simulink model "osek_apis"  (Simulink 6.0)
settings: Solver=FixedStepDiscrete  StartTime=0.0  StopTime=10.0  RelTol=1e-3
undefined symbols (not defined in the file or in its folder): D4, D5, green, red
libraries: oseklib x5, simulink x3, osekdrivers x2
settings Model: Creator=jcarrick  LastModifiedBy=jcarrick  ProdHWDeviceType=Motorola PowerPC
settings SolverCC: PositivePriorityOrder=on
settings DataIOCC: SignalLoggingName=sigsOut
settings OptimizationCC: InlineParams=on  InlineInvariantSignals=off  OptimizeModelRefInitCode=on  LifeSpan=1
settings DebuggingCC: CheckExecutionContextPreStartOutputMsg=on  CheckExecutionContextRuntimeOutputMsg=on  SolverPrmCheckMsg=none
settings HardwareCC: ProdEndianess=BigEndian  ProdHWDeviceType=Motorola PowerPC
settings RTWCC: SystemTargetFile=osekworks.tlc  GenCodeOnly=on  TemplateMakefile=osek_default_tmf  GenerateReport=on  RetainRTWFile=on  ProcessScript=osekworks_make_rtw_hook  IncludeHyperlinkInReport=on  LaunchReport=on
settings CodeAppCC: IgnoreCustomStorageClasses=off
settings STFCustomTargetCC: TargetFcnLib=ansi_tfl_tmw.mat  GenFloatMathFcnCalls=ANSI_C  ModelReferenceCompliant=off  CombineOutputUpdateFcns=on  SuppressErrorStatus=on  ERTCustomFileBanners=on  SystemTargetFile=osekworks.tlc  ForcedBaseTarget=off
settings ERTTargetCC: TargetFcnLib=ansi_tfl_tmw.mat  GenFloatMathFcnCalls=ANSI_C  ModelReferenceCompliant=off  SuppressErrorStatus=on  SupportContinuousTime=on  SupportNonInlinedSFcns=on  RootIOFormat=Individual Arguments  ERTCustomFileTemplate=osek_file_process.tlc  InitialValueSource=Model
settings CustomProperty: DataType=RTWOptions_EnumType__toolbox_rtw_targets_osek_osek_osekworks_bspName  Value=phycore555
settings EnumStrPairs: String=axiomcmd565
settings SFSimCC: SFSimApplyToAllLibs=on  SFSimBuildMode=Incremental

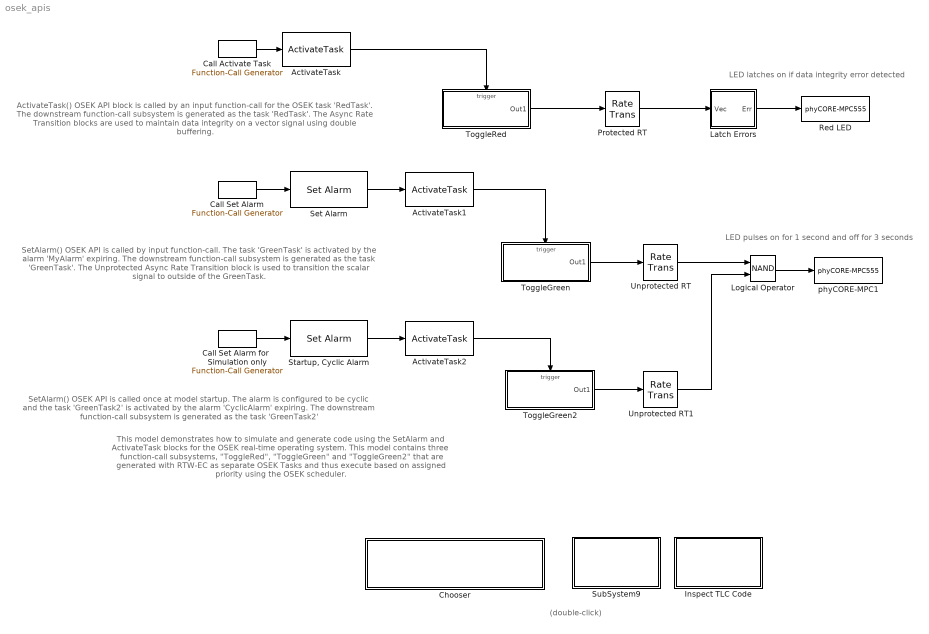
== system osek_apis ==
  note: This model demonstrates how to simulate and generate code using the SetAlarm and ActivateTask blocks
      | for the OSEK real-time operating system. This model contains three function-call subsystems, "ToggleRed",
      | "ToggleGreen" and "ToggleGreen2" that are generated with RTW-EC as separate OSEK Tasks and thus
      | execute based on assigned priority using the OSEK scheduler.
  note: (double-click)
  note: ActivateTask() OSEK API block is called by an input
      | function-call for the OSEK task 'RedTask'. The downstream
      | function-call subsystem is generated as the task 'RedTask'.
      | The Async Rate Transition blocks are used to maintain
      | data integrity on a vector signal using double buffering.
  note: SetAlarm() OSEK API is called by input function-call. The task
      | 'GreenTask' is activated by the alarm 'MyAlarm' expiring. The
      | downstream function-call subsystem is generated as the task 'GreenTask'.
      | The Unprotected Async Rate Transition block is used to transition the
      | scalar signal to outside of the GreenTask.
  note: SetAlarm() OSEK API is called once at model startup. The alarm
      | is configured to be cyclic and the task 'GreenTask2' is activated by
      | the alarm 'CyclicAlarm' expiring. The downstream function-call
      | subsystem is generated as the task 'GreenTask2'
  note: LED pulses on for 1 second and off for 3 seconds
  note: LED latches on if data integrity error detected
  ActivateTask : oseklib/ActivateTask  taskName=RedTask  taskPriority=10  taskStackSize=1000  taskSchedule=FULL
  ActivateTask1 : oseklib/ActivateTask  taskName=GreenTask  taskPriority=31  taskStackSize=100  taskSchedule=NON
  ActivateTask2 : oseklib/ActivateTask  taskName=GreenTask2  taskPriority=32  taskStackSize=100  taskSchedule=NON
  Call Activate Task : simulink/Ports & Subsystems/Function-Call Generator  sample_time=1  numberOfIterations=1
  Call Set Alarm : simulink/Ports & Subsystems/Function-Call Generator  sample_time=1  numberOfIterations=1
  Call Set Alarm for  Simulation only : simulink/Ports & Subsystems/Function-Call Generator  sample_time=2  numberOfIterations=1
  Chooser : Subsystem  LoadFcn=|  PropExecContextAcrossSSBoundary=on  mask{stf=osekworks.tlc}
      | x = osek.prefs.load('osek');                               
      | Implementation = lower(x.Implementation);                  
      | clear x;                                                   
      | switch Implementation                                      
      |  case {'proosek','osekworks'}                              
      |   osek_choose_imp([Implementation,'.tlc']);                
      |   set_param(gcb,'MaskValueString',[Implementation,'.tlc']);
      |  otherwise                                                 
      |   error(['Unrecognized implementation: ' Implementation]); 
      | end                                                        
      | clear Implementation;
      mask prompts: stf "Implementation"
      mask help: Choose OSEK System Target File
      mask init:
      | osek_choose_imp(stf)
      mask StyleString: popup(osekworks.tlc|proosek.tlc)
      mask Display: disp(['Choose System Target File:\nCurrently set to "' strtok(get_param(gcs,'rtwsystemtargetfile')) '"'])
  Inspect TLC Code : Subsystem  PropExecContextAcrossSSBoundary=on
      mask Display: disp('Inspect\nBlock\nTLC Code')
  Latch Errors : Subsystem  TreatAsAtomicUnit=on  PropExecContextAcrossSSBoundary=on
      settings: RTWSystemCode=Function
  Logical Operator : Logic  Operator=NAND  AllPortsSameDT=off
  Protected RT : RateTransition  Deterministic=off  OutPortSampleTime=.25
  Red LED : osekdrivers/phyCORE-MPC555  ledChoice=D4(red)
  Set Alarm : oseklib/Set Alarm  alarmName=MyAlarm  alarmIncr=1  alarmType=Relative  alarmPlacement=off  alarmCyclic=0
  "Startup, Cyclic Alarm" : oseklib/Set Alarm  alarmName=cyclicAlarm  alarmIncr=1  alarmType=Relative  alarmPlacement=on  alarmCyclic=8
  SubSystem9 : Subsystem  PropExecContextAcrossSSBoundary=on
      settings: OpenFcn=rtwbuild('osek_apis');
      mask Display: disp('Generate\nCode')
  ToggleGreen : Subsystem  TreatAsAtomicUnit=on  PropExecContextAcrossSSBoundary=on
      settings: RTWSystemCode=Function
  ToggleGreen2 : Subsystem  TreatAsAtomicUnit=on  PropExecContextAcrossSSBoundary=on
      settings: RTWSystemCode=Function
  ToggleRed : Subsystem  TreatAsAtomicUnit=on  PropExecContextAcrossSSBoundary=on
      settings: RTWSystemCode=Function
  Unprotected RT : RateTransition  Integrity=off  OutPortSampleTime=1
  Unprotected RT1 : RateTransition  Integrity=off  OutPortSampleTime=1
  phyCORE-MPC1 : osekdrivers/phyCORE-MPC555  ledChoice=D5(green)
  wires:
  ActivateTask/1 -> ToggleRed/Trigger
  ToggleRed/1(Out1) -> Protected RT/1
  Call Activate Task/1 -> ActivateTask/1
  Latch Errors/1(Err) -> Red LED/1
  Protected RT/1 -> Latch Errors/1(Vec)
  Set Alarm/1 -> ActivateTask1/1
  Call Set Alarm/1 -> Set Alarm/1
  ActivateTask1/1 -> ToggleGreen/Trigger
  ToggleGreen/1(Out1) -> Unprotected RT/1
  "Startup, Cyclic Alarm"/1 -> ActivateTask2/1
  Call Set Alarm for  Simulation only/1 -> "Startup, Cyclic Alarm"/1
  ActivateTask2/1 -> ToggleGreen2/Trigger
  ToggleGreen2/1(Out1) -> Unprotected RT1/1
  Unprotected RT/1 -> Logical Operator/1
  Unprotected RT1/1 -> Logical Operator/2
  Logical Operator/1 -> phyCORE-MPC1/1

== system osek_apis/Chooser ==

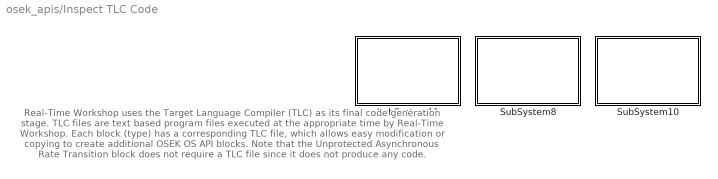
== system osek_apis/Inspect TLC Code ==
  note: Real-Time Workshop uses the Target Language Compiler (TLC) as its final code generation stage.
      | TLC files are text based program files executed at the appropriate time by Real-Time Workshop.
      | Each block (type) has a corresponding TLC file, which allows easy modification or copying to create
      | additional OSEK OS API blocks. Note that the Unprotected Asynchronous Rate Transition block does
      | not require a TLC file since it does not produce any code.
  SubSystem10 : Subsystem  PropExecContextAcrossSSBoundary=on
      settings: OpenFcn=edit(fullfile(matlabroot,'toolbox','rtw','targets','osek','blocks','osekdbuffer.tlc'));
      mask Display: disp('Inspect\nAsync Rate\nTransition\nTLC File')
  SubSystem11 : Subsystem  PropExecContextAcrossSSBoundary=on
      settings: OpenFcn=edit(fullfile(matlabroot,'toolbox','rtw','targets','osek','blocks','osektask.tlc'));
      mask Display: disp('Inspect\nActivateTask\nTLC File')
  SubSystem8 : Subsystem  PropExecContextAcrossSSBoundary=on
      settings: OpenFcn=edit(fullfile(matlabroot,'toolbox','rtw','targets','osek','blocks','oseksetalarm.tlc'));
      mask Display: disp('Inspect\nSetAlarm\nTLC File')

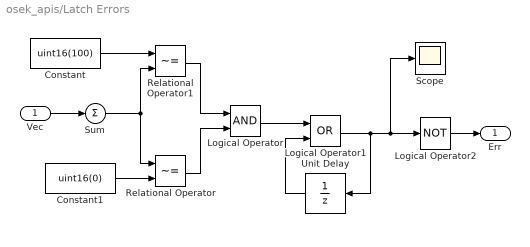
== system osek_apis/Latch Errors ==
  Vec : Inport  LatchInput=off
  Constant : Constant  Value=uint16(100)
  Constant1 : Constant  Value=uint16(0)
  Logical Operator : Logic  AllPortsSameDT=off
  Logical Operator1 : Logic  Operator=OR  AllPortsSameDT=off
  Logical Operator2 : Logic  Operator=NOT  AllPortsSameDT=off
  Relational Operator : RelationalOperator  Operator=~=
  Relational Operator1 : RelationalOperator  Operator=~=
  Scope : Scope
  Sum : Sum  Inputs=1  SaturateOnIntegerOverflow=on
  Unit Delay : UnitDelay  Orientation=left  SampleTime=-1
  Err : Outport
  wires:
  Vec/1 -> Sum/1
  Constant/1 -> Relational Operator1/1
  Constant1/1 -> Relational Operator/2
  Relational Operator1/1 -> Logical Operator/1
  Relational Operator/1 -> Logical Operator/2
  Logical Operator/1 -> Logical Operator1/1
  Logical Operator1/1 -> Unit Delay/1, Logical Operator2/1, Scope/1
  Unit Delay/1 -> Logical Operator1/2
  Logical Operator2/1 -> Err/1
  Sum/1 -> Relational Operator/1, Relational Operator1/2

== system osek_apis/SubSystem9 ==

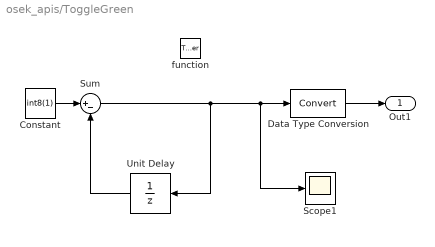
== system osek_apis/ToggleGreen ==
  function : TriggerPort  TriggerType=function-call
  Constant : Constant  Value=int8(1)
  Data Type Conversion : DataTypeConversion  SaturateOnIntegerOverflow=on  RndMeth=Zero
  Scope1 : Scope
      settings: SaveName=ScopeData2
  Sum : Sum  Inputs=|+-  SaturateOnIntegerOverflow=on
  Unit Delay : UnitDelay  Orientation=left  SampleTime=-1
  Out1 : Outport
  wires:
  Unit Delay/1 -> Sum/2
  Constant/1 -> Sum/1
  Sum/1 -> Unit Delay/1, Data Type Conversion/1, Scope1/1
  Data Type Conversion/1 -> Out1/1

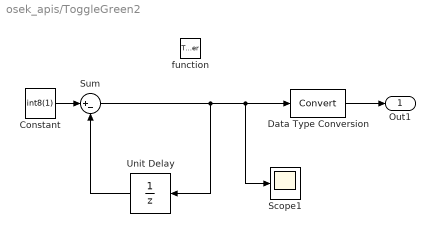
== system osek_apis/ToggleGreen2 ==
  function : TriggerPort  TriggerType=function-call
  Constant : Constant  Value=int8(1)
  Data Type Conversion : DataTypeConversion  SaturateOnIntegerOverflow=on  RndMeth=Zero
  Scope1 : Scope
      settings: SaveName=ScopeData3
  Sum : Sum  Inputs=|+-  SaturateOnIntegerOverflow=on
  Unit Delay : UnitDelay  Orientation=left  SampleTime=-1
  Out1 : Outport
  wires:
  Data Type Conversion/1 -> Out1/1
  Sum/1 -> Unit Delay/1, Data Type Conversion/1, Scope1/1
  Constant/1 -> Sum/1
  Unit Delay/1 -> Sum/2

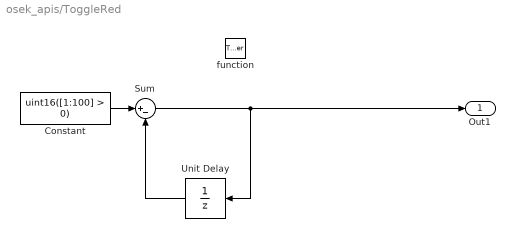
== system osek_apis/ToggleRed ==
  function : TriggerPort  TriggerType=function-call
  Constant : Constant  Value=uint16([1:100] > 0)  OutDataTypeMode=uint16
  Sum : Sum  Inputs=|+-  SaturateOnIntegerOverflow=on
  Unit Delay : UnitDelay  Orientation=left  SampleTime=-1
  Out1 : Outport
  wires:
  Sum/1 -> Unit Delay/1, Out1/1
  Constant/1 -> Sum/1
  Unit Delay/1 -> Sum/2

== system osek_apis/Inspect TLC Code/SubSystem10 ==

== system osek_apis/Inspect TLC Code/SubSystem11 ==

== system osek_apis/Inspect TLC Code/SubSystem8 ==
